simulink model "pedulumpid"  (Simulink 8.3)
settings: Solver=ode45  StartTime=0.0  StopTime=10  RelTol=1e-3
settings Model: Creator=Mr-Yu  LastModifiedBy=Administrator
settings DataIOCC: SignalLoggingName=sigsOut
settings OptimizationCC: ExpressionDepthLimit=2147483647  InitFltsAndDblsToZero=on
settings DebuggingCC: SaveWithParameterizedLinksMsg=none  SignalResolutionControl=TryResolveAllWithWarning  SolverPrmCheckMsg=none  MultiTaskDSMMsg=warning  MultiTaskCondExecSysMsg=none  FcnCallInpInsideContextMsg=UseLocalSettings
settings HardwareCC: TargetUnknown=on
settings RTWCC: IncludeERTFirstTime=on
settings GRTTargetCC: TargetFcnLib=ansi_tfl_tmw.mat

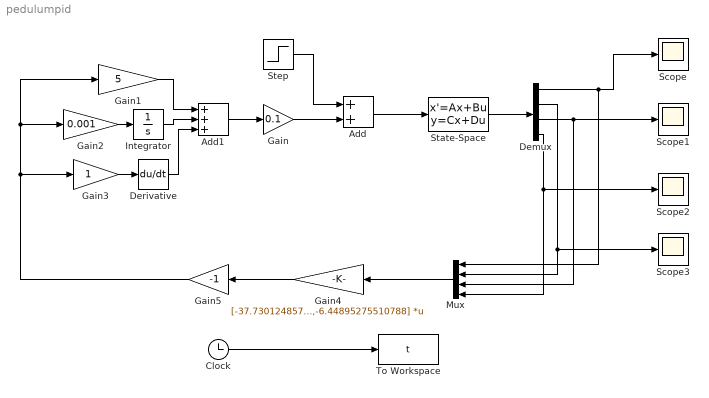
== system pedulumpid ==
  Add : Sum
  Add1 : Sum  Inputs=+++
  Clock : Clock
  Demux : Demux
  Derivative : Derivative
  Gain : Gain  Gain=0.1
  Gain1 : Gain  Gain=5
  Gain2 : Gain  Gain=0.001
  Gain3 : Gain
  Gain4 : Gain  Gain=[-37.7301248571561,-6.11083393673725,-4.90186428572187,-6.44895275510788]  Multiplication=Matrix(K*u)
  Gain5 : Gain  Gain=-1
  Integrator : Integrator
  Mux : Mux
  Scope{,1..3} (4 alike) : Scope
      Scope settings: TimeRange=10  YMin=0  YMax=1.5e+25
      Scope2 settings: SaveName=ScopeData2
      Scope3 settings: SaveName=ScopeData3
  State-Space : StateSpace  A=[0,1,0,0;51.5789473684211,0,0,0.526315789473684;0,0,0,1;-7.73684210526316,0,0,-0.178947368421053]  B=[0;-5.26315789473684;0;1.78947368421053]  C=[1 0 0 0;0 1 0 0;0 0 1 0;0 0 0 1]  D=[0;0;0;0]  X0=0
  Step : Step  Time=0  After=0.25  SampleTime=0
  To Workspace : ToWorkspace  VariableName=t  SampleTime=-1
  wires:
  Add/1 -> State-Space/1
  Step/1 -> Add/1
  Gain/1 -> Add/2
  Add1/1 -> Gain/1
  Gain1/1 -> Add1/1
  Gain2/1 -> Integrator/1
  Integrator/1 -> Add1/2
  Gain3/1 -> Derivative/1
  Derivative/1 -> Add1/3
  Mux/1 -> Gain4/1
  Gain4/1 -> Gain5/1
  Gain5/1 -> Gain3/1, Gain2/1, Gain1/1
  State-Space/1 -> Demux/1
  Demux/1 -> Scope/1, Mux/1
  Demux/3 -> Scope1/1, Mux/3
  Demux/2 -> Scope3/1, Mux/2
  Demux/4 -> Scope2/1, Mux/4
  Clock/1 -> To Workspace/1
